simulink model "Ex5_2"  (R2016b)
settings: Solver=VariableStepAuto  StartTime=0.0  StopTime=1000  RelTol=1e-3
values from neighbouring files (symbols this model uses):
  J = 0.05    [Ex5_2_init.m]    (also in Ex5_3_init.m; Home54_init.m = 0.5; homepart51.m)
  L_r_al_bet0 = [M*real(I_s) + L_r*real(I_r); M*imag(I_s)+L_r*imag(I_r)]    [Ex5_2_init.m]
  L_s_al_bet0 = [L_s*real(I_s)+M*real(I_r); L_s*imag(I_s)+M*imag(I_r)]    [Ex5_2_init.m]
  M = 0.082    [Ex5_2_init.m]    (also in Ex5_3_init.m = 0.0082; homepart51.m)
  p = 1    [Ex5_2_init.m]    (also in Ex5_3_init.m; Home54_init.m; homepart51.m)
  R_r = 0.3    [Ex5_2_init.m]    (also in Ex5_3_init.m = 0.003)
  R_s = 0.3    [Ex5_2_init.m]    (also in Ex5_3_init.m)
  Ur = 0    [Ex5_2_init.m]
  Us = sqrt(2)*Uphase    [Ex5_2_init.m]    (also in Ex5_3_init.m = Us_rat/Ws_rat * ws)
  wm = 2910/60*2*pi    (= 304.734487398)    [Ex5_2_init.m]
  ws = 50*2*pi    (= 314.159265359)    [Ex5_2_init.m]    (also in Ex5_3_init.m)
libraries: powerlib_meascontrol x1
settings Model: Creator=Niels  LastModifiedBy=Niels

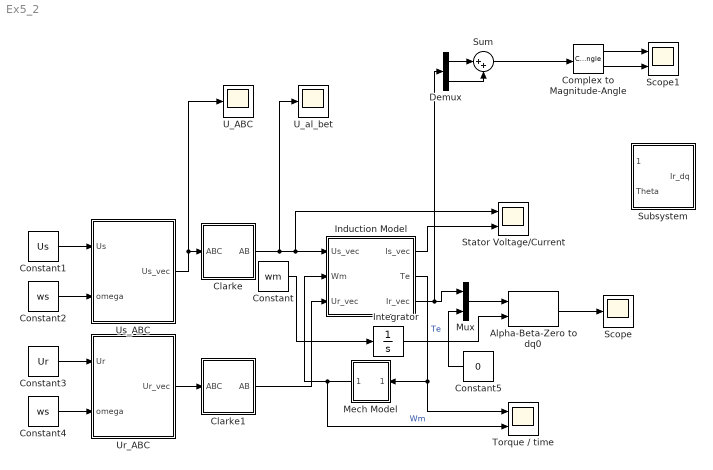
== system Ex5_2 ==
  Alpha-Beta-Zero to dq0 : powerlib_meascontrol/Transformations/Alpha-Beta-Zero to dq0  Alignment=90 degrees behind phase A axis
  Clarke : Subsystem
  Clarke1 : Subsystem
  Complex to Magnitude-Angle : ComplexToMagnitudeAngle
  Constant : Constant  Value=wm
  Constant1 : Constant  Value=Us
  Constant2 : Constant  Value=ws
  Constant3 : Constant  Value=Ur
  Constant4 : Constant  Value=ws
  Constant5 : Constant  Value=0
  Demux : Demux  Outputs=2
  Induction Model : Subsystem
  Integrator : Integrator
  Mech Model : Subsystem
  Mux : Mux  Inputs=2
  Scope : Scope
  Scope1 : Scope  NumInputPorts=2
  "Stator Voltage/Current " : Scope  NumInputPorts=2
  Subsystem : Subsystem
  Sum : Sum  Inputs=|++
  Torque / time : Scope  NumInputPorts=2
  "U_ABC " : Scope
  U_al_bet : Scope
  Ur_ABC : Subsystem
  Us_ABC : Subsystem
  wires:
  Mech Model/1(wm) -> Induction Model/2(Wm), Torque / time/2  "Wm"
  Constant1/1 -> Us_ABC/1(Us)
  Constant2/1 -> Us_ABC/2(omega)
  Constant3/1 -> Ur_ABC/1(Ur)
  Constant4/1 -> Ur_ABC/2(omega)
  Us_ABC/1(Us_vec) -> "U_ABC "/1, Clarke/1(ABC)
  Ur_ABC/1(Ur_vec) -> Clarke1/1(ABC)
  Clarke/1(AB) -> U_al_bet/1, "Stator Voltage/Current "/1, Induction Model/1(Us_vec)
  Clarke1/1(AB) -> Induction Model/3(Ur_vec)
  Induction Model/1(Is_vec) -> "Stator Voltage/Current "/2
  Induction Model/2(Te) -> Mech Model/1(Te), Torque / time/1  "Te"
  Alpha-Beta-Zero to dq0/1 -> Scope/1
  Constant/1 -> Integrator/1
  Mux/1 -> Alpha-Beta-Zero to dq0/1
  Constant5/1 -> Mux/2
  Integrator/1 -> Alpha-Beta-Zero to dq0/2
  Induction Model/3(Ir_vec) -> Demux/1, Mux/1
  Complex to Magnitude-Angle/1 -> Scope1/1
  Complex to Magnitude-Angle/2 -> Scope1/2
  Demux/1 -> Sum/1
  Demux/2 -> Sum/2
  Sum/1 -> Complex to Magnitude-Angle/1

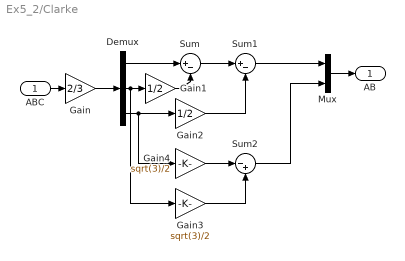
== system Ex5_2/Clarke ==
  ABC : Inport
  Demux : Demux  Outputs=3
  Gain : Gain  Gain=2/3
  Gain1 : Gain  Gain=1/2
  Gain2 : Gain  Gain=1/2
  Gain3 : Gain  Gain=sqrt(3)/2
  Gain4 : Gain  Gain=sqrt(3)/2
  Mux : Mux  Inputs=2
  Sum : Sum  Inputs=|+-
  Sum1 : Sum  Inputs=|+-
  Sum2 : Sum  Inputs=|-+
  AB : Outport
  wires:
  ABC/1 -> Gain/1
  Mux/1 -> AB/1
  Gain/1 -> Demux/1
  Demux/1 -> Sum/1
  Demux/2 -> Gain3/1, Gain1/1
  Gain1/1 -> Sum/2
  Sum/1 -> Sum1/1
  Sum1/1 -> Mux/1
  Demux/3 -> Gain4/1, Gain2/1
  Gain2/1 -> Sum1/2
  Gain4/1 -> Sum2/1
  Gain3/1 -> Sum2/2
  Sum2/1 -> Mux/2

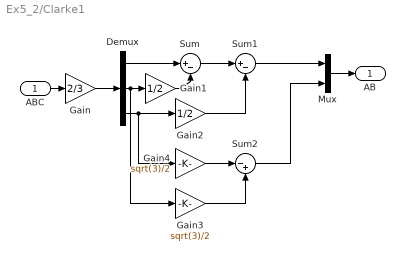
== system Ex5_2/Clarke1 ==
  ABC : Inport
  Demux : Demux  Outputs=3
  Gain : Gain  Gain=2/3
  Gain1 : Gain  Gain=1/2
  Gain2 : Gain  Gain=1/2
  Gain3 : Gain  Gain=sqrt(3)/2
  Gain4 : Gain  Gain=sqrt(3)/2
  Mux : Mux  Inputs=2
  Sum : Sum  Inputs=|+-
  Sum1 : Sum  Inputs=|+-
  Sum2 : Sum  Inputs=|-+
  AB : Outport
  wires:
  ABC/1 -> Gain/1
  Mux/1 -> AB/1
  Gain/1 -> Demux/1
  Demux/1 -> Sum/1
  Demux/2 -> Gain3/1, Gain1/1
  Gain1/1 -> Sum/2
  Sum/1 -> Sum1/1
  Sum1/1 -> Mux/1
  Demux/3 -> Gain4/1, Gain2/1
  Gain2/1 -> Sum1/2
  Gain4/1 -> Sum2/1
  Gain3/1 -> Sum2/2
  Sum2/1 -> Mux/2

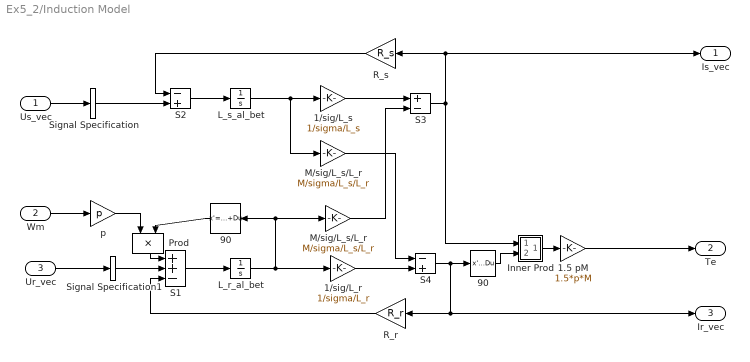
== system Ex5_2/Induction Model ==
  Us_vec : Inport
  Wm : Inport  Port=2
  Ur_vec : Inport  Port=3
  1.5 pM : Gain  Gain=1.5*p*M  SaturateOnIntegerOverflow=on  OutDataTypeStr=Inherit: Same as input  ParamDataTypeStr=Inherit: Same as input
  1/sig/L_r : Gain  Gain=1/sigma/L_r  SaturateOnIntegerOverflow=on  OutDataTypeStr=Inherit: Same as input  ParamDataTypeStr=Inherit: Same as input
  "1/sig/L_s " : Gain  Gain=1/sigma/L_s  SaturateOnIntegerOverflow=on  OutDataTypeStr=Inherit: Same as input  ParamDataTypeStr=Inherit: Same as input
  90 : StateSpace  A=[]  B=[]  C=[]  D=K  X0=0  mask(Matrix gain){K=[0 -1;1 0]}
      mask prompts: K "Gain matrix:"
      mask help: Matrix Gain.
      mask Help: Multiplies input vector by entered matrix to produce output vector (y=Au).
      mask Display: disp('K')
  "90 " : StateSpace  A=[]  B=[]  C=[]  D=K  X0=0  mask(Matrix gain){K=[0 -1;1 0]}
      mask prompts: K "Gain matrix:"
      mask help: Matrix Gain.
      mask Help: Multiplies input vector by entered matrix to produce output vector (y=Au).
      mask Display: disp('K')
  Inner Prod : Subsystem  mask(Dot Product){}
      mask help:
      | Inner (dot) product.
      | y=sum(u1.*u2)
      mask Help: Computes the inner (dot) product of the inputs: sum(u1.*u2).  The inputs are vectors of the same length. Output is a scalar.
      mask Display: disp('.\n')
  L_r_al_bet : Integrator  InitialCondition=L_r_al_bet0
  L_s_al_bet : Integrator  InitialCondition=L_s_al_bet0
  M/sig/L_s/L_r : Gain  Gain=M/sigma/L_s/L_r  SaturateOnIntegerOverflow=on  OutDataTypeStr=Inherit: Same as input  ParamDataTypeStr=Inherit: Same as input
  "M/sig/L_s/L_r " : Gain  Gain=M/sigma/L_s/L_r  SaturateOnIntegerOverflow=on  OutDataTypeStr=Inherit: Same as input  ParamDataTypeStr=Inherit: Same as input
  Prod : Product  SaturateOnIntegerOverflow=on  RndMeth=Zero  InputSameDT=on  OutDataTypeStr=Inherit: Same as first input
  R_r : Gain  Gain=R_r  SaturateOnIntegerOverflow=on  OutDataTypeStr=Inherit: Same as input  ParamDataTypeStr=Inherit: Same as input
  R_s : Gain  Gain=R_s  SaturateOnIntegerOverflow=on  OutDataTypeStr=Inherit: Same as input  ParamDataTypeStr=Inherit: Same as input
  S1 : Sum  Inputs=++-  SaturateOnIntegerOverflow=on  InputSameDT=on  OutDataTypeStr=Inherit: Same as first input
  S2 : Sum  Inputs=-+  SaturateOnIntegerOverflow=on  InputSameDT=on  OutDataTypeStr=Inherit: Same as first input
  S3 : Sum  Inputs=+-  SaturateOnIntegerOverflow=on  InputSameDT=on  OutDataTypeStr=Inherit: Same as first input
  S4 : Sum  Inputs=-+  SaturateOnIntegerOverflow=on  InputSameDT=on  OutDataTypeStr=Inherit: Same as first input
  Signal Specification : SignalSpecification  Dimensions=[2 1]
  Signal Specification1 : SignalSpecification  Dimensions=[2 1]
  p : Gain  Gain=p  SaturateOnIntegerOverflow=on  OutDataTypeStr=Inherit: Same as input  ParamDataTypeStr=Inherit: Same as input
  Is_vec : Outport
  Te : Outport  Port=2
  Ir_vec : Outport  Port=3
  wires:
  Wm/1 -> p/1
  S4/1 -> Ir_vec/1, R_r/1, "90 "/1
  S3/1 -> Is_vec/1, R_s/1, Inner Prod/1(in_1)
  p/1 -> Prod/1
  Us_vec/1 -> Signal Specification/1
  R_r/1 -> S1/3
  L_s_al_bet/1 -> "1/sig/L_s "/1, M/sig/L_s/L_r/1
  S2/1 -> L_s_al_bet/1
  90/1 -> Prod/2
  Ur_vec/1 -> Signal Specification1/1
  M/sig/L_s/L_r/1 -> S4/1
  L_r_al_bet/1 -> 1/sig/L_r/1, "M/sig/L_s/L_r "/1, 90/1
  R_s/1 -> S2/1
  1.5 pM/1 -> Te/1
  "1/sig/L_s "/1 -> S3/1
  S1/1 -> L_r_al_bet/1
  "M/sig/L_s/L_r "/1 -> S3/2
  1/sig/L_r/1 -> S4/2
  Inner Prod/1(out_1) -> 1.5 pM/1
  Prod/1 -> S1/1
  "90 "/1 -> Inner Prod/2(in_2)
  Signal Specification/1 -> S2/2
  Signal Specification1/1 -> S1/2

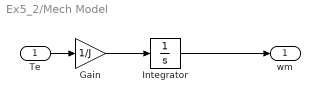
== system Ex5_2/Mech Model ==
  Te : Inport
  Gain : Gain  Gain=1/J
  Integrator : Integrator
  wm : Outport
  wires:
  Te/1 -> Gain/1
  Gain/1 -> Integrator/1
  Integrator/1 -> wm/1

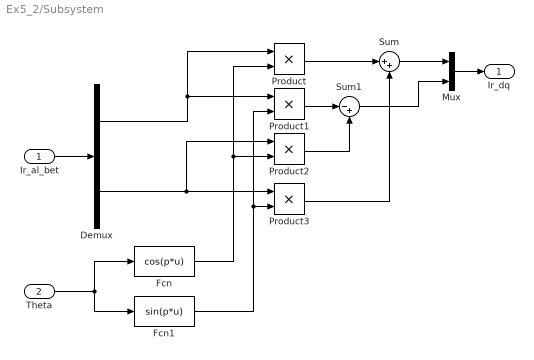
== system Ex5_2/Subsystem ==
  Ir_al_bet : Inport
  Theta : Inport  Port=2
  Demux : Demux  Outputs=2
  Fcn : Fcn  Expr=cos(p*u)
  Fcn1 : Fcn  Expr=sin(p*u)
  Mux : Mux  Inputs=2
  Product{,1..3} (4 alike) : Product
  Sum : Sum  Inputs=|++
  Sum1 : Sum  Inputs=|-+
  Ir_dq : Outport
  wires:
  Theta/1 -> Fcn/1, Fcn1/1
  Ir_al_bet/1 -> Demux/1
  Demux/1 -> Product1/1, Product/1
  Demux/2 -> Product2/1, Product3/1
  Fcn/1 -> Product2/2, Product/2
  Fcn1/1 -> Product3/2, Product1/2
  Product/1 -> Sum/1
  Product3/1 -> Sum/2
  Sum/1 -> Mux/1
  Product1/1 -> Sum1/1
  Product2/1 -> Sum1/2
  Sum1/1 -> Mux/2
  Mux/1 -> Ir_dq/1

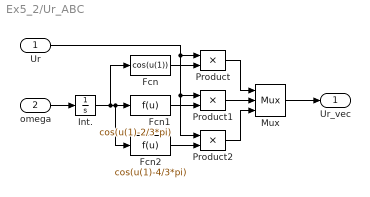
== system Ex5_2/Ur_ABC ==
  Ur : Inport
  omega : Inport  Port=2
  Fcn : Fcn  Expr=cos(u(1))
  Fcn1 : Fcn  Expr=cos(u(1)-2/3*pi)
  Fcn2 : Fcn  Expr=cos(u(1)-4/3*pi)
  Int. : Integrator
  Mux : Mux  Inputs=3
  Product : Product  SaturateOnIntegerOverflow=on  RndMeth=Zero  InputSameDT=on  OutDataTypeStr=Inherit: Same as first input
  Product1 : Product  SaturateOnIntegerOverflow=on  RndMeth=Zero  InputSameDT=on  OutDataTypeStr=Inherit: Same as first input
  Product2 : Product  SaturateOnIntegerOverflow=on  RndMeth=Zero  InputSameDT=on  OutDataTypeStr=Inherit: Same as first input
  Ur_vec : Outport
  wires:
  Fcn2/1 -> Product2/2
  Int./1 -> Fcn1/1, Fcn2/1, Fcn/1
  Fcn1/1 -> Product1/2
  Product/1 -> Mux/1
  Product2/1 -> Mux/3
  Mux/1 -> Ur_vec/1
  Product1/1 -> Mux/2
  omega/1 -> Int./1
  Ur/1 -> Product/1, Product1/1, Product2/1
  Fcn/1 -> Product/2

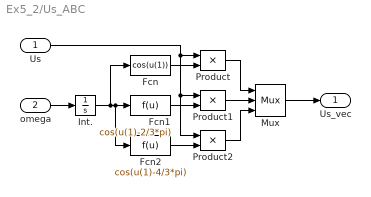
== system Ex5_2/Us_ABC ==
  Us : Inport
  omega : Inport  Port=2
  Fcn : Fcn  Expr=cos(u(1))
  Fcn1 : Fcn  Expr=cos(u(1)-2/3*pi)
  Fcn2 : Fcn  Expr=cos(u(1)-4/3*pi)
  Int. : Integrator
  Mux : Mux  Inputs=3
  Product : Product  SaturateOnIntegerOverflow=on  RndMeth=Zero  InputSameDT=on  OutDataTypeStr=Inherit: Same as first input
  Product1 : Product  SaturateOnIntegerOverflow=on  RndMeth=Zero  InputSameDT=on  OutDataTypeStr=Inherit: Same as first input
  Product2 : Product  SaturateOnIntegerOverflow=on  RndMeth=Zero  InputSameDT=on  OutDataTypeStr=Inherit: Same as first input
  Us_vec : Outport
  wires:
  Fcn2/1 -> Product2/2
  Fcn1/1 -> Product1/2
  Product/1 -> Mux/1
  Product2/1 -> Mux/3
  Mux/1 -> Us_vec/1
  Product1/1 -> Mux/2
  omega/1 -> Int./1
  Us/1 -> Product/1, Product1/1, Product2/1
  Fcn/1 -> Product/2
  Int./1 -> Fcn1/1, Fcn2/1, Fcn/1

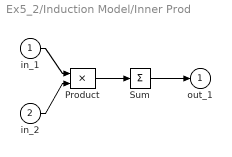
== system Ex5_2/Induction Model/Inner Prod ==
  in_1 : Inport
  in_2 : Inport  Port=2
  Product : Product  SaturateOnIntegerOverflow=on  RndMeth=Zero  InputSameDT=on  OutDataTypeStr=Inherit: Same as first input
  Sum : Sum  Inputs=+  SaturateOnIntegerOverflow=on  InputSameDT=on  OutDataTypeStr=Inherit: Same as first input
  out_1 : Outport
  wires:
  in_2/1 -> Product/2
  in_1/1 -> Product/1
  Product/1 -> Sum/1
  Sum/1 -> out_1/1
